simulink model "arm_forward_kinematics_func"  (R2023a)
settings: Solver=VariableStepAuto  StartTime=0.0  StopTime=10.0  RelTol=1e-3
settings Model: Creator=Marwa  LastModifiedBy=Nada Tamer
settings ModelReferenceCC: EnableRefExpFcnMdlSchedulingChecks=on

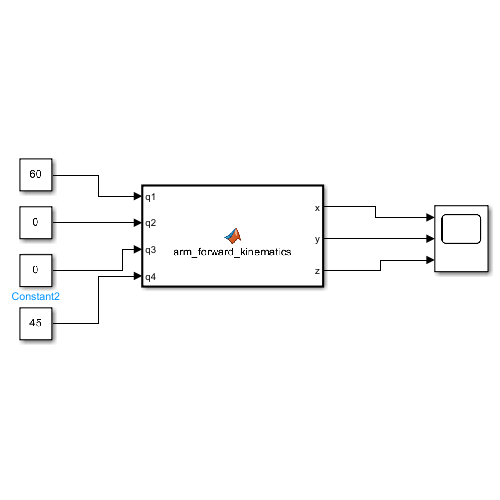
[thumbnail: Simulink's stored preview of the top-level diagram]
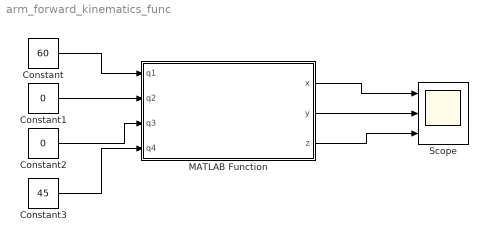
== system arm_forward_kinematics_func ==
  Constant : Constant  Value=60
  Constant1 : Constant  Value=0
  Constant2 : Constant  Value=0
  Constant3 : Constant  Value=45
  MATLAB Function : MATLAB Function  TreatAsAtomicUnit=on
  Scope : Scope  NumInputPorts=3
  wires:
  Constant3/1 -> MATLAB Function/4(q4)
  Constant2/1 -> MATLAB Function/3(q3)
  Constant/1 -> MATLAB Function/1(q1)
  Constant1/1 -> MATLAB Function/2(q2)
  MATLAB Function/1(x) -> Scope/1
  MATLAB Function/2(y) -> Scope/2
  MATLAB Function/3(z) -> Scope/3

== matlab function arm_forward_kinematics_func/MATLAB Function ==
  data: q1 input; x output; q2 input; q3 input; q4 input; y output; z output
function [x,y,z] = arm_forward_kinematics(q1,q2,q3,q4)
% l1 = 1;
% l2 = 2;
% l3 = 3;
% l4 = 4;
l1 = 0.0288811487749;%old: 0.0291
l2 = 0.02659997;%old: 0.04406
l3 = 0.12240002;%old: 0.10416
l4 = 0.15;%old: 0.15444

X = [l4*cos((pi*q1)/180)*sin((pi*(q2-90))/180)*sin((pi*(q4-90))/180)-l4*cos((pi*(q4-90))/180)*(sin((pi*q1)/180)*sin((pi*(q3-90))/180)-cos((pi*q1)/180)*cos((pi*(q2-90))/180)*cos((pi*(q3-90))/180))-cos((pi*q1)/180)*sin((pi*(q2-90))/180)*(l2+l3);
    l4*cos((pi*(q4-90))/180)*(cos((pi*q1)/180)*sin((pi*(q3-90))/180)+sin((pi*q1)/180)*cos((pi*(q2-90))/180)*cos((pi*(q3-90))/180))-sin((pi*q1)/180)*sin((pi*(q2-90))/180)*(l2+l3)+l4*sin((pi*q1)/180)*sin((pi*(q2-90))/180)*sin((pi*(q4-90))/180);
    l4*cos((pi*(q2-90))/180)*sin((pi*(q4-90))/180)-cos((pi*(q2-90))/180)*(l2+l3)-l1-l4*cos((pi*(q3-90))/180)*cos((pi*(q4-90))/180)*sin((pi*(q2-90))/180)];
      
x = X(1,1);
y = X(2,1);
z = X(3,1);
